simulink model "ITCG_2D_salvo_attack"  (R2023b)
settings: Solver=ode4  StartTime=0.0  StopTime=45  FixedStep=1/100  RelTol=1e-3
libraries: simulink x4, simulink_extras x1
settings Model: Creator=Administrator  LastModifiedBy=Administrator
settings DebuggingCC: UnderSpecifiedDimensionMsg=warning

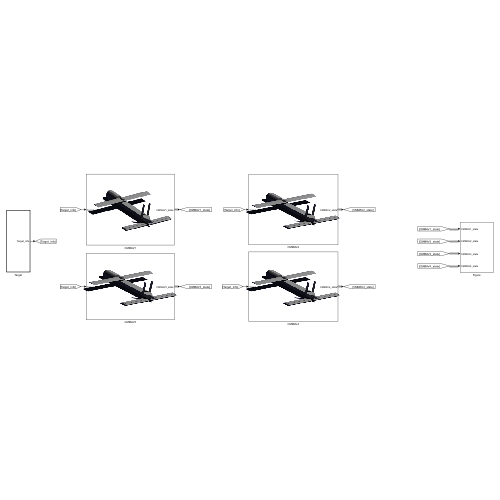
[thumbnail: Simulink's stored preview of the top-level diagram]
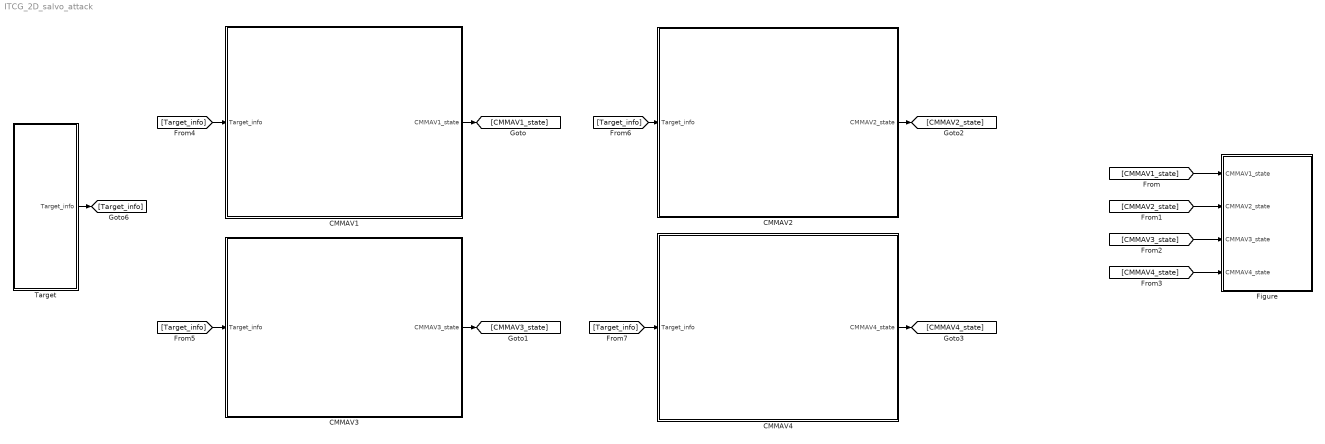
== system ITCG_2D_salvo_attack ==
  CMMAV1 : Subsystem
      mask Display: image('그림5.svg');
  CMMAV2 : Subsystem
  CMMAV3 : Subsystem
  CMMAV4 : Subsystem
  Figure : Subsystem
  Target : Subsystem  TreatAsAtomicUnit=on
  wires:
  [CMMAV1_state] -> Figure/1(CMMAV1_state)
  CMMAV1/1(CMMAV1_state) -> [CMMAV1_state]
  CMMAV3/1(CMMAV3_state) -> [CMMAV3_state]
  CMMAV2/1(CMMAV2_state) -> [CMMAV2_state]
  CMMAV4/1(CMMAV4_state) -> [CMMAV4_state]
  [CMMAV2_state] -> Figure/2(CMMAV2_state)
  [CMMAV3_state] -> Figure/3(CMMAV3_state)
  [CMMAV4_state] -> Figure/4(CMMAV4_state)
  Target/1(Target_info) -> [Target_info]
  [Target_info] -> CMMAV1/1(Target_info)
  [Target_info] -> CMMAV3/1(Target_info)
  [Target_info] -> CMMAV2/1(Target_info)
  [Target_info] -> CMMAV4/1(Target_info)

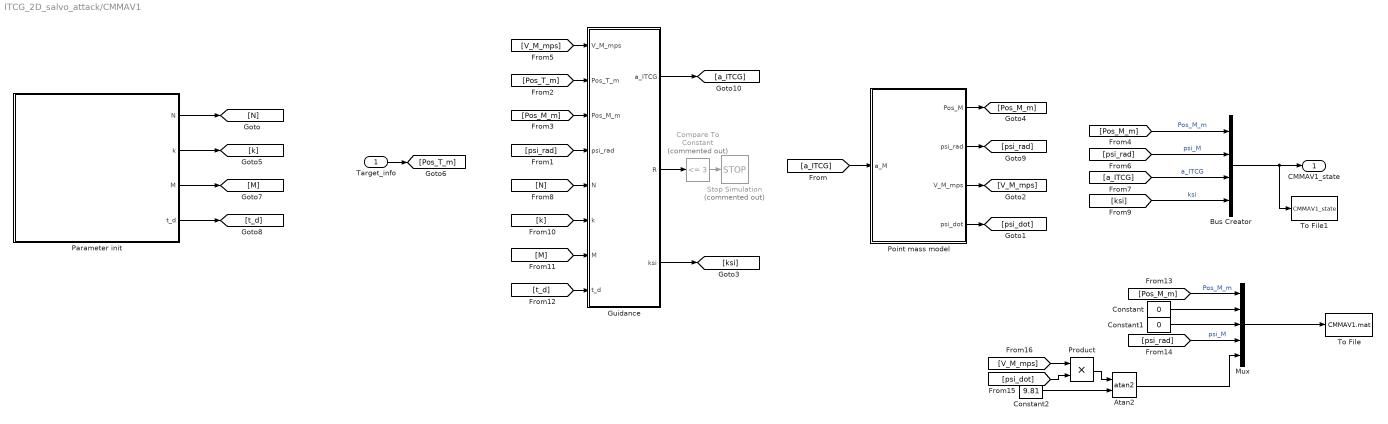
== system ITCG_2D_salvo_attack/CMMAV1 ==
  Target_info : Inport
  Atan2 : Trigonometry  Operator=atan2
  Bus Creator : BusCreator  Inputs=4
  Compare To Constant : simulink/Logic and Bit Operations/Compare To Constant  Commented=on  relop=<=  const=3  OutDataTypeStr=boolean
  Constant : Constant  Value=0
  Constant1 : Constant  Value=0
  Constant2 : Constant  Value=9.81
  Guidance : Subsystem
  Mux : Mux  Inputs=5
  Parameter init : Subsystem
  Point mass model : Subsystem
  Product : Product
  Stop Simulation : Stop  Commented=on
  To File : ToFile  Filename=CMMAV1.mat
  To File1 : ToFile  Filename=CMMAV1_state
  CMMAV1_state : Outport
  wires:
  Point mass model/2(psi_rad) -> [psi_rad]
  [M] -> Guidance/7(M)
  [k] -> Guidance/6(k)
  [Pos_M_m] -> Guidance/3(Pos_M_m)
  Target_info/1 -> [Pos_T_m]
  [N] -> Guidance/5(N)
  [a_ITCG] -> Point mass model/1(a_M)
  [Pos_T_m] -> Guidance/2(Pos_T_m)
  Guidance/2(R) -> Compare To Constant/1
  Point mass model/1(Pos_M) -> [Pos_M_m]
  [V_M_mps] -> Guidance/1(V_M_mps)
  [t_d] -> Guidance/8(t_d)
  Compare To Constant/1 -> Stop Simulation/1
  [psi_rad] -> Guidance/4(psi_rad)
  Guidance/1(a_ITCG) -> [a_ITCG]
  Point mass model/3(V_M_mps) -> [V_M_mps]
  Guidance/3(ksi) -> [ksi]
  Parameter init/3(M) -> [M]
  Parameter init/4(t_d) -> [t_d]
  Parameter init/2(k) -> [k]
  Parameter init/1(N) -> [N]
  [Pos_M_m] -> Bus Creator/1  "Pos_M_m"
  [psi_rad] -> Bus Creator/2  "psi_M"
  [a_ITCG] -> Bus Creator/3  "a_ITCG"
  [ksi] -> Bus Creator/4  "ksi"
  Bus Creator/1 -> To File1/1, CMMAV1_state/1
  [Pos_M_m] -> Mux/1  "Pos_M_m"
  Constant/1 -> Mux/2
  Constant1/1 -> Mux/3
  Point mass model/4(psi_dot) -> [psi_dot]
  Constant2/1 -> Atan2/2
  [psi_dot] -> Product/2
  [V_M_mps] -> Product/1
  Product/1 -> Atan2/1
  Atan2/1 -> Mux/5
  Mux/1 -> To File/1
  [psi_rad] -> Mux/4  "psi_M"

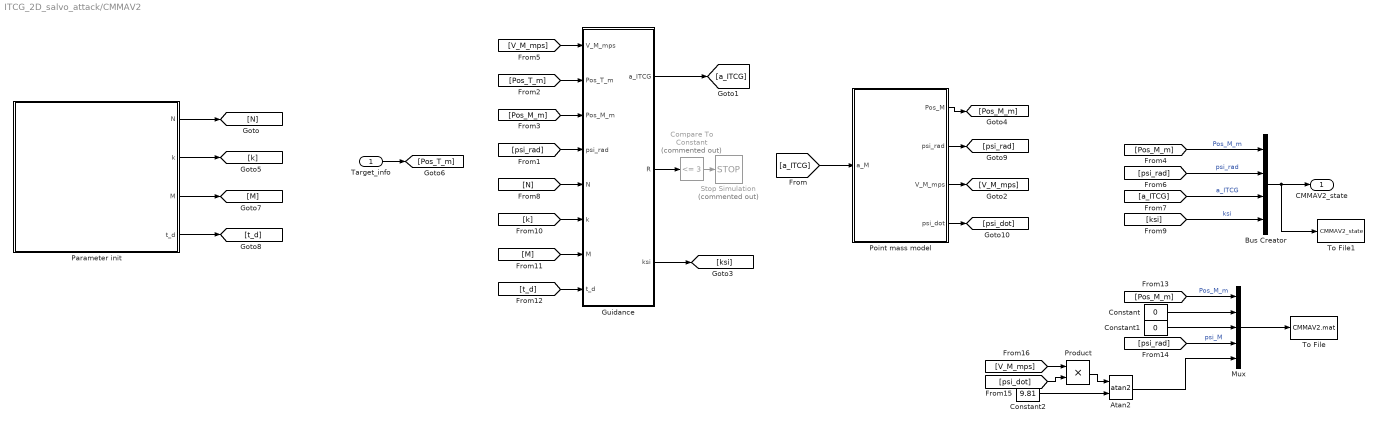
== system ITCG_2D_salvo_attack/CMMAV2 ==
  Target_info : Inport
  Atan2 : Trigonometry  Operator=atan2
  Bus Creator : BusCreator  Inputs=4
  Compare To Constant : simulink/Logic and Bit Operations/Compare To Constant  Commented=on  relop=<=  const=3  OutDataTypeStr=boolean
  Constant : Constant  Value=0
  Constant1 : Constant  Value=0
  Constant2 : Constant  Value=9.81
  Guidance : Subsystem
  Mux : Mux  Inputs=5
  Parameter init : Subsystem
  Point mass model : Subsystem
  Product : Product
  Stop Simulation : Stop  Commented=on
  To File : ToFile  Filename=CMMAV2.mat
  To File1 : ToFile  Filename=CMMAV2_state
  CMMAV2_state : Outport
  wires:
  Point mass model/2(psi_rad) -> [psi_rad]
  [M] -> Guidance/7(M)
  [k] -> Guidance/6(k)
  [Pos_M_m] -> Guidance/3(Pos_M_m)
  [N] -> Guidance/5(N)
  [a_ITCG] -> Point mass model/1(a_M)
  [Pos_T_m] -> Guidance/2(Pos_T_m)
  Guidance/2(R) -> Compare To Constant/1
  Point mass model/1(Pos_M) -> [Pos_M_m]
  [V_M_mps] -> Guidance/1(V_M_mps)
  [t_d] -> Guidance/8(t_d)
  Compare To Constant/1 -> Stop Simulation/1
  [psi_rad] -> Guidance/4(psi_rad)
  Guidance/1(a_ITCG) -> [a_ITCG]
  Point mass model/3(V_M_mps) -> [V_M_mps]
  Guidance/3(ksi) -> [ksi]
  Parameter init/1(N) -> [N]
  Parameter init/2(k) -> [k]
  Parameter init/3(M) -> [M]
  Parameter init/4(t_d) -> [t_d]
  [psi_rad] -> Bus Creator/2  "psi_rad"
  [ksi] -> Bus Creator/4  "ksi"
  [Pos_M_m] -> Bus Creator/1  "Pos_M_m"
  [a_ITCG] -> Bus Creator/3  "a_ITCG"
  Mux/1 -> To File/1
  [V_M_mps] -> Product/1
  Constant2/1 -> Atan2/2
  Product/1 -> Atan2/1
  Atan2/1 -> Mux/5
  Constant1/1 -> Mux/3
  [psi_rad] -> Mux/4  "psi_M"
  Constant/1 -> Mux/2
  [psi_dot] -> Product/2
  [Pos_M_m] -> Mux/1  "Pos_M_m"
  Point mass model/4(psi_dot) -> [psi_dot]
  Target_info/1 -> [Pos_T_m]
  Bus Creator/1 -> To File1/1, CMMAV2_state/1

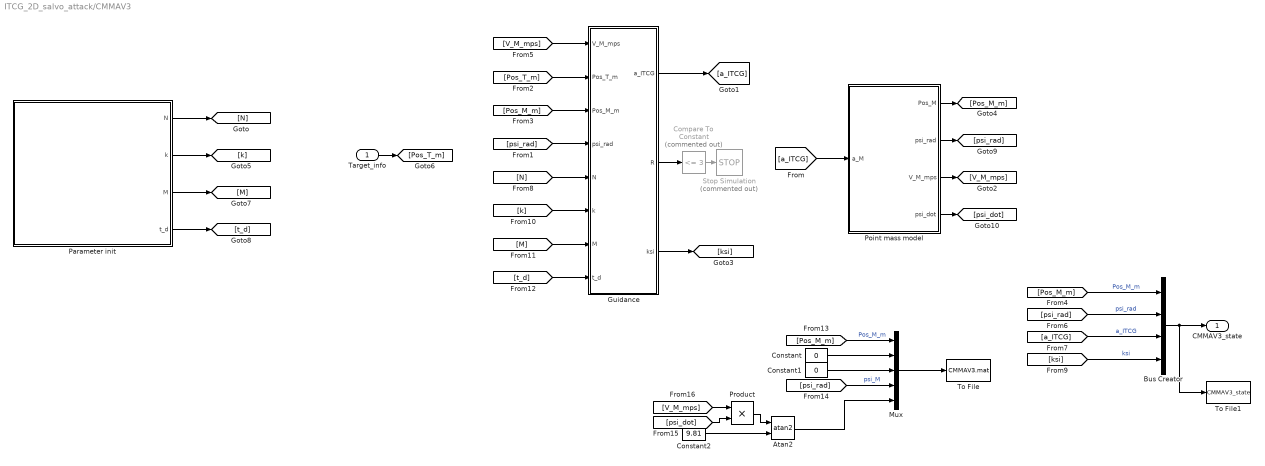
== system ITCG_2D_salvo_attack/CMMAV3 ==
  Target_info : Inport
  Atan2 : Trigonometry  Operator=atan2
  Bus Creator : BusCreator  Inputs=4
  Compare To Constant : simulink/Logic and Bit Operations/Compare To Constant  Commented=on  relop=<=  const=3  OutDataTypeStr=boolean
  Constant : Constant  Value=0
  Constant1 : Constant  Value=0
  Constant2 : Constant  Value=9.81
  Guidance : Subsystem
  Mux : Mux  Inputs=5
  Parameter init : Subsystem
  Point mass model : Subsystem
  Product : Product
  Stop Simulation : Stop  Commented=on
  To File : ToFile  Filename=CMMAV3.mat
  To File1 : ToFile  Filename=CMMAV3_state
  CMMAV3_state : Outport
  wires:
  Point mass model/2(psi_rad) -> [psi_rad]
  [M] -> Guidance/7(M)
  [k] -> Guidance/6(k)
  [Pos_M_m] -> Guidance/3(Pos_M_m)
  Target_info/1 -> [Pos_T_m]
  [N] -> Guidance/5(N)
  [a_ITCG] -> Point mass model/1(a_M)
  [Pos_T_m] -> Guidance/2(Pos_T_m)
  Guidance/2(R) -> Compare To Constant/1
  Point mass model/1(Pos_M) -> [Pos_M_m]
  [V_M_mps] -> Guidance/1(V_M_mps)
  [t_d] -> Guidance/8(t_d)
  Compare To Constant/1 -> Stop Simulation/1
  [psi_rad] -> Guidance/4(psi_rad)
  Guidance/1(a_ITCG) -> [a_ITCG]
  Point mass model/3(V_M_mps) -> [V_M_mps]
  Guidance/3(ksi) -> [ksi]
  Parameter init/1(N) -> [N]
  Parameter init/2(k) -> [k]
  Parameter init/3(M) -> [M]
  Parameter init/4(t_d) -> [t_d]
  [psi_rad] -> Bus Creator/2  "psi_rad"
  [ksi] -> Bus Creator/4  "ksi"
  [Pos_M_m] -> Bus Creator/1  "Pos_M_m"
  [a_ITCG] -> Bus Creator/3  "a_ITCG"
  Mux/1 -> To File/1
  [V_M_mps] -> Product/1
  Constant2/1 -> Atan2/2
  Product/1 -> Atan2/1
  Atan2/1 -> Mux/5
  Constant1/1 -> Mux/3
  [psi_rad] -> Mux/4  "psi_M"
  Constant/1 -> Mux/2
  [psi_dot] -> Product/2
  [Pos_M_m] -> Mux/1  "Pos_M_m"
  Point mass model/4(psi_dot) -> [psi_dot]
  Bus Creator/1 -> CMMAV3_state/1, To File1/1

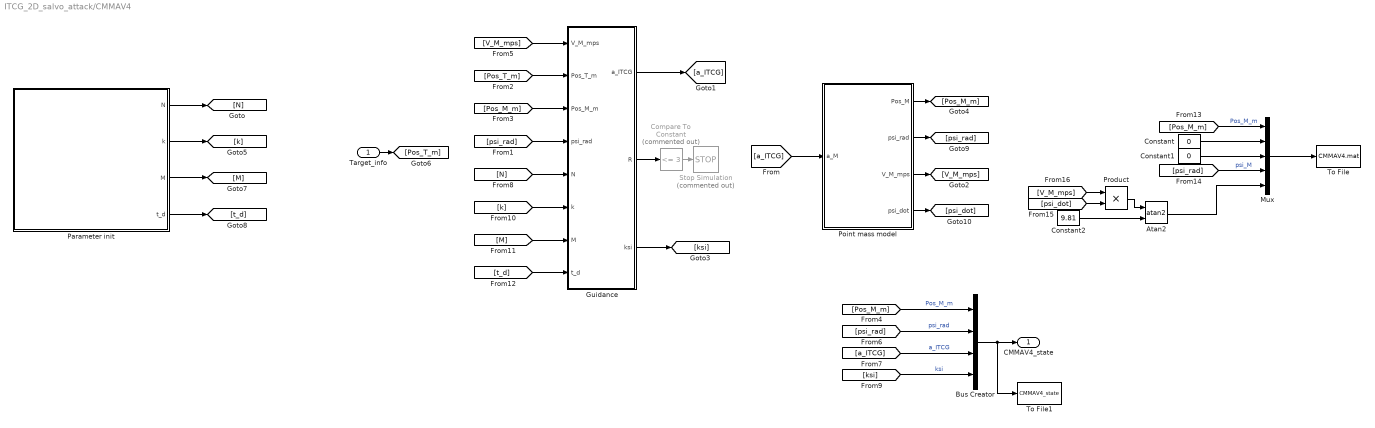
== system ITCG_2D_salvo_attack/CMMAV4 ==
  Target_info : Inport
  Atan2 : Trigonometry  Operator=atan2
  Bus Creator : BusCreator  Inputs=4
  Compare To Constant : simulink/Logic and Bit Operations/Compare To Constant  Commented=on  relop=<=  const=3  OutDataTypeStr=boolean
  Constant : Constant  Value=0
  Constant1 : Constant  Value=0
  Constant2 : Constant  Value=9.81
  Guidance : Subsystem
  Mux : Mux  Inputs=5
  Parameter init : Subsystem
  Point mass model : Subsystem
  Product : Product
  Stop Simulation : Stop  Commented=on
  To File : ToFile  Filename=CMMAV4.mat
  To File1 : ToFile  Filename=CMMAV4_state
  CMMAV4_state : Outport
  wires:
  Point mass model/2(psi_rad) -> [psi_rad]
  [M] -> Guidance/7(M)
  [k] -> Guidance/6(k)
  [Pos_M_m] -> Guidance/3(Pos_M_m)
  Target_info/1 -> [Pos_T_m]
  [N] -> Guidance/5(N)
  [a_ITCG] -> Point mass model/1(a_M)
  [Pos_T_m] -> Guidance/2(Pos_T_m)
  Guidance/2(R) -> Compare To Constant/1
  Point mass model/1(Pos_M) -> [Pos_M_m]
  [V_M_mps] -> Guidance/1(V_M_mps)
  [t_d] -> Guidance/8(t_d)
  Compare To Constant/1 -> Stop Simulation/1
  [psi_rad] -> Guidance/4(psi_rad)
  Guidance/1(a_ITCG) -> [a_ITCG]
  Point mass model/3(V_M_mps) -> [V_M_mps]
  Guidance/3(ksi) -> [ksi]
  Parameter init/1(N) -> [N]
  Parameter init/2(k) -> [k]
  Parameter init/3(M) -> [M]
  Parameter init/4(t_d) -> [t_d]
  [psi_rad] -> Bus Creator/2  "psi_rad"
  [ksi] -> Bus Creator/4  "ksi"
  [Pos_M_m] -> Bus Creator/1  "Pos_M_m"
  [a_ITCG] -> Bus Creator/3  "a_ITCG"
  Mux/1 -> To File/1
  [V_M_mps] -> Product/1
  Constant2/1 -> Atan2/2
  Product/1 -> Atan2/1
  Atan2/1 -> Mux/5
  Constant1/1 -> Mux/3
  [psi_rad] -> Mux/4  "psi_M"
  Constant/1 -> Mux/2
  [psi_dot] -> Product/2
  [Pos_M_m] -> Mux/1  "Pos_M_m"
  Point mass model/4(psi_dot) -> [psi_dot]
  Bus Creator/1 -> To File1/1, CMMAV4_state/1

== system ITCG_2D_salvo_attack/Figure ==
  note: Figure
  note: Input parameter
  CMMAV1_state : Inport
  CMMAV2_state : Inport  Port=2
  CMMAV3_state : Inport  Port=3
  CMMAV4_state : Inport  Port=4
  Bus Selector{,1..3} (4 alike) : BusSelector  OutputSignals=Pos_M_m
  Demux{1..4} (4 alike) : Demux  Outputs=2
  Figure : MATLAB Function  TreatAsAtomicUnit=on
  To Workspace : ToWorkspace  VariableName=CMMAV1_state  SampleTime=-1
  To Workspace1 : ToWorkspace  VariableName=CMMAV2_state  SampleTime=-1
  To Workspace2 : ToWorkspace  VariableName=CMMAV3_state  SampleTime=-1
  To Workspace3 : ToWorkspace  VariableName=CMMAV4_state  SampleTime=-1
  wires:
  [CMMAV1_x] -> Figure/1(CMMAV1_x)
  [CMMAV1_y] -> Figure/2(CMMAV1_y)
  [CMMAV2_x] -> Figure/3(CMMAV2_x)
  [CMMAV2_y] -> Figure/4(CMMAV2_y)
  CMMAV1_state/1 -> Bus Selector/1
  Bus Selector/1 -> To Workspace/1, Demux1/1  "<Pos_M_m>"
  Demux1/1 -> [CMMAV1_x]
  Demux1/2 -> [CMMAV1_y]
  Demux2/1 -> [CMMAV2_x]
  Demux2/2 -> [CMMAV2_y]
  Bus Selector1/1 -> To Workspace1/1, Demux2/1  "<Pos_M_m>"
  CMMAV2_state/1 -> Bus Selector1/1
  Demux3/1 -> [CMMAV3_x]
  Demux3/2 -> [CMMAV3_y]
  Bus Selector2/1 -> To Workspace2/1, Demux3/1  "<Pos_M_m>"
  CMMAV3_state/1 -> Bus Selector2/1
  Demux4/1 -> [CMMAV4_x]
  Demux4/2 -> [CMMAV4_y]
  Bus Selector3/1 -> To Workspace3/1, Demux4/1  "<Pos_M_m>"
  CMMAV4_state/1 -> Bus Selector3/1
  [CMMAV3_x] -> Figure/5(CMMAV3_x)
  [CMMAV3_y] -> Figure/6(CMMAV3_y)
  [CMMAV4_x] -> Figure/7(CMMAV4_x)
  [CMMAV4_y] -> Figure/8(CMMAV4_y)

== system ITCG_2D_salvo_attack/Target ==
  Add : Sum
  Add1 : Sum
  Demux : Demux  Outputs=2
  Demux1 : Demux  Outputs=2
  Integrator : Integrator
  Integrator1 : Integrator
  Mux1 : Mux  Inputs=2
  Target Position : Constant  Value=[00;00]  VectorParams1D=off
  Target Velocity : Constant  Value=[0;0]  VectorParams1D=off
  Target_info : Outport
  wires:
  Target Velocity/1 -> Demux/1
  Target Position/1 -> Demux1/1
  Add/1 -> Mux1/1
  Add1/1 -> Mux1/2
  Mux1/1 -> Target_info/1
  Demux1/1 -> [rT_x]
  [rT_x] -> Add/1
  Demux1/2 -> [rT_Y]
  [rT_Y] -> Add1/1
  Demux/1 -> [vT_x]
  Demux/2 -> [rT_y]
  [vT_xt] -> Add/2
  [vT_yt] -> Add1/2
  [vT_x] -> Integrator/1
  [rT_y] -> Integrator1/1
  Integrator/1 -> [vT_xt]
  Integrator1/1 -> [vT_yt]

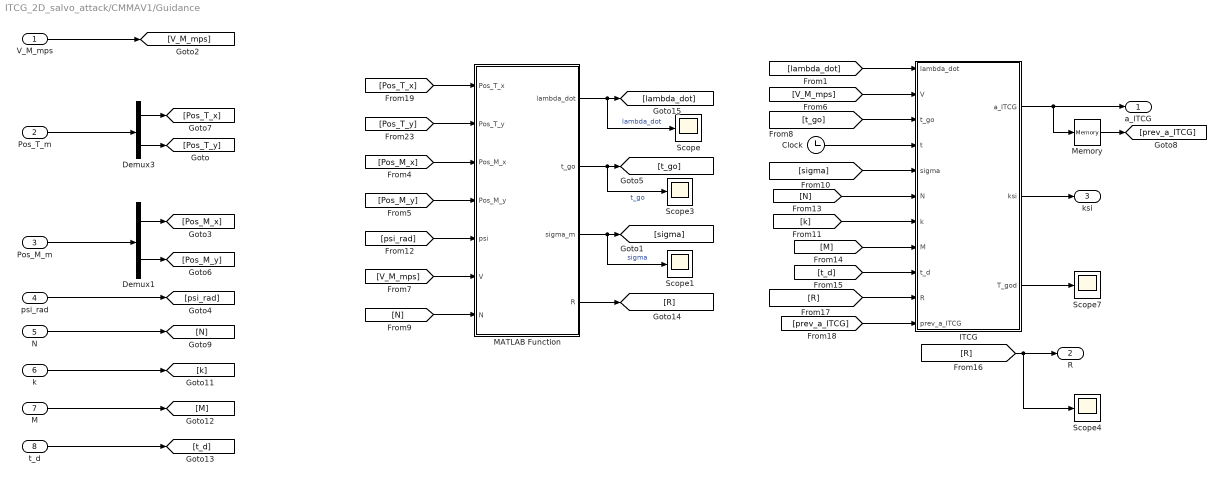
== system ITCG_2D_salvo_attack/CMMAV1/Guidance ==
  V_M_mps : Inport
  Pos_T_m : Inport  Port=2
  Pos_M_m : Inport  Port=3
  psi_rad : Inport  Port=4
  N : Inport  Port=5
  k : Inport  Port=6
  M : Inport  Port=7
  t_d : Inport  Port=8
  Clock : Clock
  Demux1 : Demux  Outputs=2
  Demux3 : Demux  Outputs=2
  ITCG : MATLAB Function  TreatAsAtomicUnit=on
  MATLAB Function : MATLAB Function  TreatAsAtomicUnit=on
  Memory : Memory
  Scope{,1,3..4,7} (5 alike) : Scope
  a_ITCG : Outport
  R : Outport  Port=2
  ksi : Outport  Port=3
  wires:
  ITCG/1(a_ITCG) -> Memory/1, a_ITCG/1
  V_M_mps/1 -> [V_M_mps]
  [V_M_mps] -> ITCG/2(V)
  [lambda_dot] -> ITCG/1(lambda_dot)
  [V_M_mps] -> MATLAB Function/6(V)
  psi_rad/1 -> [psi_rad]
  Pos_T_m/1 -> Demux3/1
  Demux3/1 -> [Pos_T_x]
  Demux1/2 -> [Pos_M_y]
  Pos_M_m/1 -> Demux1/1
  Demux1/1 -> [Pos_M_x]
  Demux3/2 -> [Pos_T_y]
  MATLAB Function/1(lambda_dot) -> [lambda_dot], Scope/1  "lambda_dot"
  MATLAB Function/2(t_go) -> Scope3/1, [t_go]  "t_go"
  Clock/1 -> ITCG/4(t)
  [Pos_M_x] -> MATLAB Function/3(Pos_M_x)
  [Pos_M_y] -> MATLAB Function/4(Pos_M_y)
  [Pos_T_x] -> MATLAB Function/1(Pos_T_x)
  [Pos_T_y] -> MATLAB Function/2(Pos_T_y)
  [psi_rad] -> MATLAB Function/5(psi)
  MATLAB Function/3(sigma_m) -> Scope1/1, [sigma]  "sigma"
  [t_go] -> ITCG/3(t_go)
  [sigma] -> ITCG/5(sigma)
  ITCG/2(ksi) -> ksi/1
  N/1 -> [N]
  t_d/1 -> [t_d]
  M/1 -> [M]
  k/1 -> [k]
  [N] -> MATLAB Function/7(N)
  [N] -> ITCG/6(N)
  [k] -> ITCG/7(k)
  [M] -> ITCG/8(M)
  [t_d] -> ITCG/9(t_d)
  MATLAB Function/4(R) -> [R]
  [R] -> Scope4/1, R/1
  [R] -> ITCG/10(R)
  Memory/1 -> [prev_a_ITCG]
  [prev_a_ITCG] -> ITCG/11(prev_a_ITCG)
  ITCG/3(T_god) -> Scope7/1

== system ITCG_2D_salvo_attack/CMMAV1/Parameter init ==
  Constant : Constant  Value=3
  Constant1 : Constant  Value=2
  Constant2 : Constant  Value=10
  Constant3 : Constant  Value=30
  N : Outport
  k : Outport  Port=2
  M : Outport  Port=3
  t_d : Outport  Port=4
  wires:
  Constant/1 -> N/1
  Constant1/1 -> k/1
  Constant2/1 -> M/1
  Constant3/1 -> t_d/1

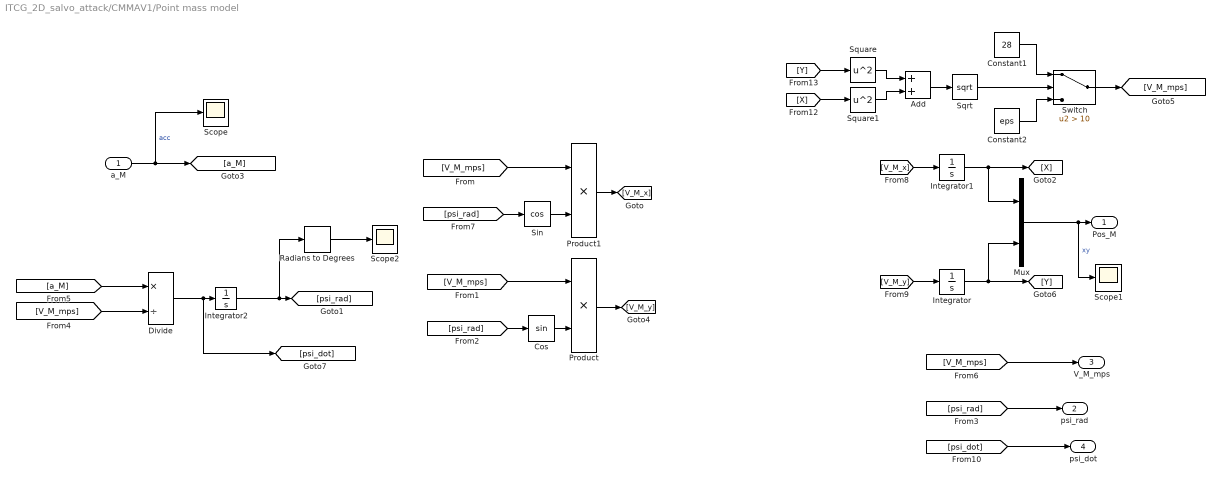
== system ITCG_2D_salvo_attack/CMMAV1/Point mass model ==
  a_M : Inport
  Add : Sum
  Constant1 : Constant  Value=28
  Constant2 : Constant  Value=eps
  Cos : Trigonometry
  Divide : Product  Inputs=*/
  Integrator : Integrator  InitialCondition=500
  Integrator1 : Integrator  InitialCondition=300
  Integrator2 : Integrator  InitialCondition=0*pi/180
  Mux : Mux  Inputs=2
  Product : Product
  Product1 : Product
  Radians to Degrees : simulink_extras/Transformations/Radians to Degrees
  Scope : Scope
  Scope1 : Scope
  Scope2 : Scope
  Sin : Trigonometry  Operator=cos
  Sqrt : Sqrt
  Square : Math  Operator=square
  Square1 : Math  Operator=square
  Switch : Switch  Criteria=u2 > Threshold  Threshold=10  SaturateOnIntegerOverflow=off  InputSameDT=off
  Pos_M : Outport
  psi_rad : Outport  Port=2
  V_M_mps : Outport  Port=3
  psi_dot : Outport  Port=4
  wires:
  [V_M_mps] -> Product1/1
  [V_M_mps] -> Product/1
  [psi_rad] -> Sin/1
  [psi_rad] -> Cos/1
  Cos/1 -> Product/2
  Sin/1 -> Product1/2
  Mux/1 -> Scope1/1, Pos_M/1  "xy"
  [psi_rad] -> psi_rad/1
  Integrator/1 -> [Y], Mux/2
  Integrator1/1 -> [X], Mux/1
  Divide/1 -> [psi_dot], Integrator2/1
  [V_M_mps] -> Divide/2
  [V_M_mps] -> V_M_mps/1
  [a_M] -> Divide/1
  a_M/1 -> Scope/1, [a_M]  "acc"
  Product1/1 -> [V_M_x]
  Product/1 -> [V_M_y]
  [V_M_x] -> Integrator1/1
  [V_M_y] -> Integrator/1
  Integrator2/1 -> Radians to Degrees/1, [psi_rad]
  Switch/1 -> [V_M_mps]
  [Y] -> Square/1
  Square1/1 -> Add/2
  Constant1/1 -> Switch/1
  Square/1 -> Add/1
  [X] -> Square1/1
  Sqrt/1 -> Switch/2
  Add/1 -> Sqrt/1
  Constant2/1 -> Switch/3
  [psi_dot] -> psi_dot/1
  Radians to Degrees/1 -> Scope2/1

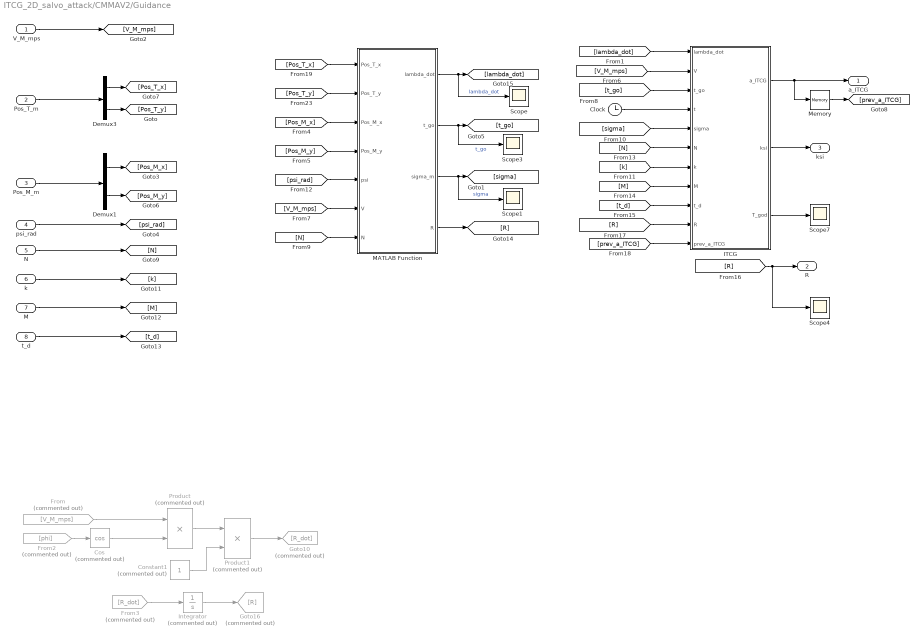
== system ITCG_2D_salvo_attack/CMMAV2/Guidance ==
  V_M_mps : Inport
  Pos_T_m : Inport  Port=2
  Pos_M_m : Inport  Port=3
  psi_rad : Inport  Port=4
  N : Inport  Port=5
  k : Inport  Port=6
  M : Inport  Port=7
  t_d : Inport  Port=8
  Clock : Clock
  Constant1 : Constant  Commented=on
  Cos : Trigonometry  Commented=on  Operator=cos
  Demux1 : Demux  Outputs=2
  Demux3 : Demux  Outputs=2
  From : From  Commented=on  GotoTag=V_M_mps
  From2 : From  Commented=on  GotoTag=phi
  From3 : From  Commented=on  GotoTag=R_dot
  Goto10 : Goto  Commented=on  GotoTag=R_dot
  Goto16 : Goto  Commented=on  GotoTag=R
  ITCG : MATLAB Function  TreatAsAtomicUnit=on
  Integrator : Integrator  Commented=on
  MATLAB Function : MATLAB Function  TreatAsAtomicUnit=on
  Memory : Memory
  Product : Product  Commented=on
  Product1 : Product  Commented=on
  Scope{,1,3..4,7} (5 alike) : Scope
  a_ITCG : Outport
  R : Outport  Port=2
  ksi : Outport  Port=3
  wires:
  ITCG/1(a_ITCG) -> Memory/1, a_ITCG/1
  V_M_mps/1 -> [V_M_mps]
  [V_M_mps] -> ITCG/2(V)
  [lambda_dot] -> ITCG/1(lambda_dot)
  [V_M_mps] -> MATLAB Function/6(V)
  psi_rad/1 -> [psi_rad]
  Pos_T_m/1 -> Demux3/1
  Demux3/1 -> [Pos_T_x]
  Demux1/2 -> [Pos_M_y]
  Pos_M_m/1 -> Demux1/1
  Demux1/1 -> [Pos_M_x]
  Demux3/2 -> [Pos_T_y]
  MATLAB Function/1(lambda_dot) -> [lambda_dot], Scope/1  "lambda_dot"
  MATLAB Function/2(t_go) -> Scope3/1, [t_go]  "t_go"
  Clock/1 -> ITCG/4(t)
  From2/1 -> Cos/1
  From/1 -> Product/1
  Cos/1 -> Product/2
  Product/1 -> Product1/1
  Constant1/1 -> Product1/2
  Product1/1 -> Goto10/1
  From3/1 -> Integrator/1
  Integrator/1 -> Goto16/1
  [Pos_M_x] -> MATLAB Function/3(Pos_M_x)
  [Pos_M_y] -> MATLAB Function/4(Pos_M_y)
  [Pos_T_x] -> MATLAB Function/1(Pos_T_x)
  [Pos_T_y] -> MATLAB Function/2(Pos_T_y)
  [psi_rad] -> MATLAB Function/5(psi)
  MATLAB Function/3(sigma_m) -> Scope1/1, [sigma]  "sigma"
  [t_go] -> ITCG/3(t_go)
  [sigma] -> ITCG/5(sigma)
  ITCG/2(ksi) -> ksi/1
  N/1 -> [N]
  t_d/1 -> [t_d]
  M/1 -> [M]
  k/1 -> [k]
  [N] -> MATLAB Function/7(N)
  [N] -> ITCG/6(N)
  [k] -> ITCG/7(k)
  [M] -> ITCG/8(M)
  [t_d] -> ITCG/9(t_d)
  MATLAB Function/4(R) -> [R]
  [R] -> Scope4/1, R/1
  [R] -> ITCG/10(R)
  Memory/1 -> [prev_a_ITCG]
  [prev_a_ITCG] -> ITCG/11(prev_a_ITCG)
  ITCG/3(T_god) -> Scope7/1

== system ITCG_2D_salvo_attack/CMMAV2/Parameter init ==
  Constant : Constant  Value=3
  Constant1 : Constant  Value=2
  Constant2 : Constant  Value=10
  Constant3 : Constant  Value=35
  N : Outport
  k : Outport  Port=2
  M : Outport  Port=3
  t_d : Outport  Port=4
  wires:
  Constant3/1 -> t_d/1
  Constant1/1 -> k/1
  Constant2/1 -> M/1
  Constant/1 -> N/1

== system ITCG_2D_salvo_attack/CMMAV2/Point mass model ==
  a_M : Inport
  Add : Sum
  Constant : Constant  Value=28
  Constant1 : Constant  Value=eps
  Cos : Trigonometry
  Divide : Product  Inputs=*/
  Integrator : Integrator  InitialCondition=500
  Integrator1 : Integrator  InitialCondition=-300
  Integrator2 : Integrator  InitialCondition=90*pi/180
  Mux : Mux  Inputs=2
  Product : Product
  Product1 : Product
  Sin : Trigonometry  Operator=cos
  Sqrt : Sqrt
  Square : Math  Operator=square
  Square1 : Math  Operator=square
  Switch : Switch  Criteria=u2 > Threshold  Threshold=10  SaturateOnIntegerOverflow=off  InputSameDT=off
  Pos_M : Outport
  psi_rad : Outport  Port=2
  V_M_mps : Outport  Port=3
  psi_dot : Outport  Port=4
  wires:
  [V_M_mps] -> Product1/1
  [V_M_mps] -> Product/1
  [psi_rad] -> Sin/1
  [psi_rad] -> Cos/1
  Cos/1 -> Product/2
  Sin/1 -> Product1/2
  Mux/1 -> Pos_M/1
  [psi_rad] -> psi_rad/1
  Integrator/1 -> [Y]
  Integrator1/1 -> [X]
  Divide/1 -> psi_dot/1, Integrator2/1
  [V_M_mps] -> Divide/2
  [V_M_mps] -> V_M_mps/1
  [a_M] -> Divide/1
  a_M/1 -> [a_M]
  Product1/1 -> [V_M_x]
  Product/1 -> [V_M_y]
  [V_M_x] -> Integrator1/1
  [V_M_y] -> Integrator/1
  Integrator2/1 -> [psi_rad]
  [Y] -> Square/1
  [X] -> Square1/1
  Square/1 -> Add/1
  Square1/1 -> Add/2
  Add/1 -> Sqrt/1
  Sqrt/1 -> Switch/2
  Constant/1 -> Switch/1
  Switch/1 -> [V_M_mps]
  Constant1/1 -> Switch/3
  [Y] -> Mux/2
  [X] -> Mux/1

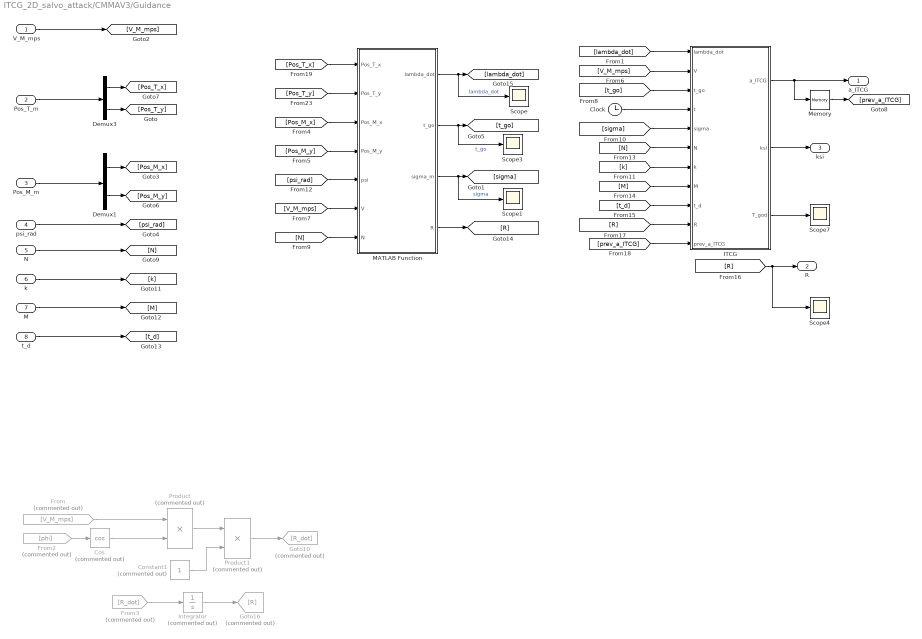
== system ITCG_2D_salvo_attack/CMMAV3/Guidance ==
  V_M_mps : Inport
  Pos_T_m : Inport  Port=2
  Pos_M_m : Inport  Port=3
  psi_rad : Inport  Port=4
  N : Inport  Port=5
  k : Inport  Port=6
  M : Inport  Port=7
  t_d : Inport  Port=8
  Clock : Clock
  Constant1 : Constant  Commented=on
  Cos : Trigonometry  Commented=on  Operator=cos
  Demux1 : Demux  Outputs=2
  Demux3 : Demux  Outputs=2
  From : From  Commented=on  GotoTag=V_M_mps
  From2 : From  Commented=on  GotoTag=phi
  From3 : From  Commented=on  GotoTag=R_dot
  Goto10 : Goto  Commented=on  GotoTag=R_dot
  Goto16 : Goto  Commented=on  GotoTag=R
  ITCG : MATLAB Function  TreatAsAtomicUnit=on
  Integrator : Integrator  Commented=on
  MATLAB Function : MATLAB Function  TreatAsAtomicUnit=on
  Memory : Memory
  Product : Product  Commented=on
  Product1 : Product  Commented=on
  Scope{,1,3..4,7} (5 alike) : Scope
  a_ITCG : Outport
  R : Outport  Port=2
  ksi : Outport  Port=3
  wires:
  ITCG/1(a_ITCG) -> Memory/1, a_ITCG/1
  V_M_mps/1 -> [V_M_mps]
  [V_M_mps] -> ITCG/2(V)
  [lambda_dot] -> ITCG/1(lambda_dot)
  [V_M_mps] -> MATLAB Function/6(V)
  psi_rad/1 -> [psi_rad]
  Pos_T_m/1 -> Demux3/1
  Demux3/1 -> [Pos_T_x]
  Demux1/2 -> [Pos_M_y]
  Pos_M_m/1 -> Demux1/1
  Demux1/1 -> [Pos_M_x]
  Demux3/2 -> [Pos_T_y]
  MATLAB Function/1(lambda_dot) -> [lambda_dot], Scope/1  "lambda_dot"
  MATLAB Function/2(t_go) -> Scope3/1, [t_go]  "t_go"
  Clock/1 -> ITCG/4(t)
  From2/1 -> Cos/1
  From/1 -> Product/1
  Cos/1 -> Product/2
  Product/1 -> Product1/1
  Constant1/1 -> Product1/2
  Product1/1 -> Goto10/1
  From3/1 -> Integrator/1
  Integrator/1 -> Goto16/1
  [Pos_M_x] -> MATLAB Function/3(Pos_M_x)
  [Pos_M_y] -> MATLAB Function/4(Pos_M_y)
  [Pos_T_x] -> MATLAB Function/1(Pos_T_x)
  [Pos_T_y] -> MATLAB Function/2(Pos_T_y)
  [psi_rad] -> MATLAB Function/5(psi)
  MATLAB Function/3(sigma_m) -> Scope1/1, [sigma]  "sigma"
  [t_go] -> ITCG/3(t_go)
  [sigma] -> ITCG/5(sigma)
  ITCG/2(ksi) -> ksi/1
  N/1 -> [N]
  t_d/1 -> [t_d]
  M/1 -> [M]
  k/1 -> [k]
  [N] -> MATLAB Function/7(N)
  [N] -> ITCG/6(N)
  [k] -> ITCG/7(k)
  [M] -> ITCG/8(M)
  [t_d] -> ITCG/9(t_d)
  MATLAB Function/4(R) -> [R]
  [R] -> Scope4/1, R/1
  [R] -> ITCG/10(R)
  Memory/1 -> [prev_a_ITCG]
  [prev_a_ITCG] -> ITCG/11(prev_a_ITCG)
  ITCG/3(T_god) -> Scope7/1

== system ITCG_2D_salvo_attack/CMMAV3/Parameter init ==
  Constant : Constant  Value=3
  Constant1 : Constant  Value=2
  Constant2 : Constant  Value=10
  Constant3 : Constant  Value=40
  N : Outport
  k : Outport  Port=2
  M : Outport  Port=3
  t_d : Outport  Port=4
  wires:
  Constant3/1 -> t_d/1
  Constant1/1 -> k/1
  Constant2/1 -> M/1
  Constant/1 -> N/1

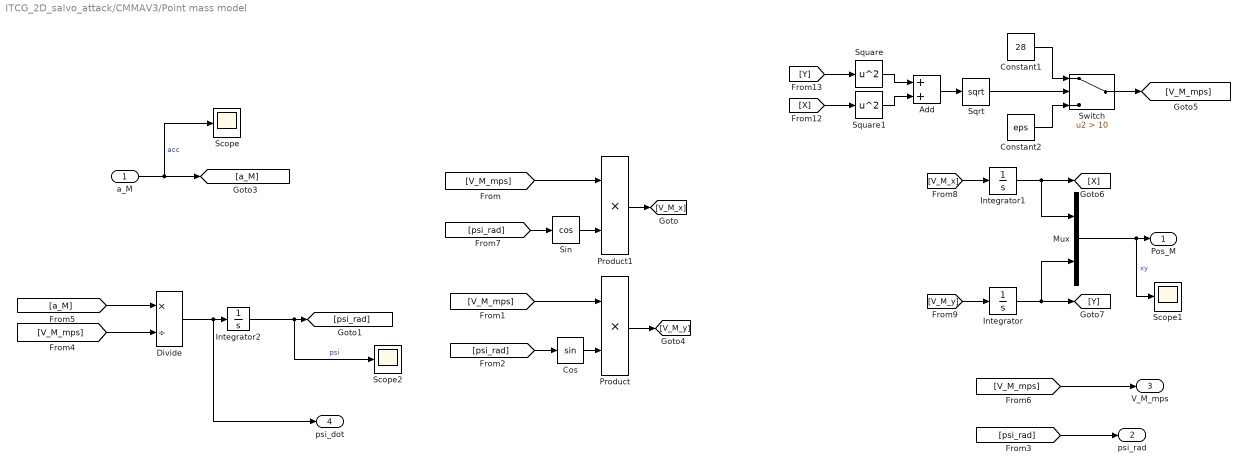
== system ITCG_2D_salvo_attack/CMMAV3/Point mass model ==
  a_M : Inport
  Add : Sum
  Constant1 : Constant  Value=28
  Constant2 : Constant  Value=eps
  Cos : Trigonometry
  Divide : Product  Inputs=*/
  Integrator : Integrator  InitialCondition=-500
  Integrator1 : Integrator  InitialCondition=300
  Integrator2 : Integrator  InitialCondition=-90*pi/180
  Mux : Mux  Inputs=2
  Product : Product
  Product1 : Product
  Scope : Scope
  Scope1 : Scope
  Scope2 : Scope
  Sin : Trigonometry  Operator=cos
  Sqrt : Sqrt
  Square : Math  Operator=square
  Square1 : Math  Operator=square
  Switch : Switch  Criteria=u2 > Threshold  Threshold=10  SaturateOnIntegerOverflow=off  InputSameDT=off
  Pos_M : Outport
  psi_rad : Outport  Port=2
  V_M_mps : Outport  Port=3
  psi_dot : Outport  Port=4
  wires:
  [V_M_mps] -> Product1/1
  [V_M_mps] -> Product/1
  [psi_rad] -> Sin/1
  [psi_rad] -> Cos/1
  Cos/1 -> Product/2
  Sin/1 -> Product1/2
  Mux/1 -> Scope1/1, Pos_M/1  "xy"
  [psi_rad] -> psi_rad/1
  Integrator/1 -> [Y], Mux/2
  Integrator1/1 -> [X], Mux/1
  Divide/1 -> psi_dot/1, Integrator2/1
  [V_M_mps] -> Divide/2
  [V_M_mps] -> V_M_mps/1
  [a_M] -> Divide/1
  a_M/1 -> Scope/1, [a_M]  "acc"
  Product1/1 -> [V_M_x]
  Product/1 -> [V_M_y]
  [V_M_x] -> Integrator1/1
  [V_M_y] -> Integrator/1
  Integrator2/1 -> Scope2/1, [psi_rad]  "psi"
  Add/1 -> Sqrt/1
  Constant2/1 -> Switch/3
  [X] -> Square1/1
  Constant1/1 -> Switch/1
  Square1/1 -> Add/2
  Sqrt/1 -> Switch/2
  Switch/1 -> [V_M_mps]
  Square/1 -> Add/1
  [Y] -> Square/1

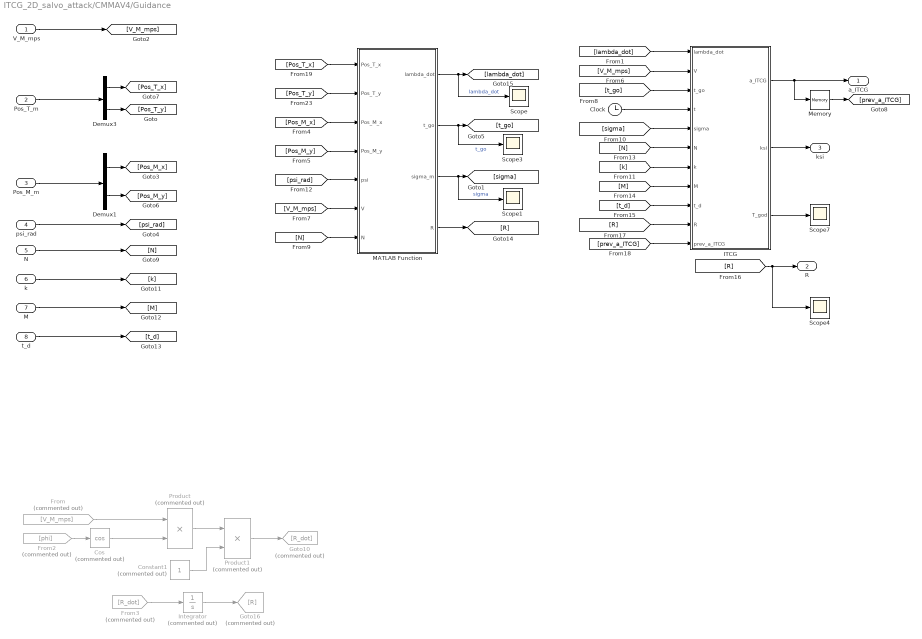
== system ITCG_2D_salvo_attack/CMMAV4/Guidance ==
  V_M_mps : Inport
  Pos_T_m : Inport  Port=2
  Pos_M_m : Inport  Port=3
  psi_rad : Inport  Port=4
  N : Inport  Port=5
  k : Inport  Port=6
  M : Inport  Port=7
  t_d : Inport  Port=8
  Clock : Clock
  Constant1 : Constant  Commented=on
  Cos : Trigonometry  Commented=on  Operator=cos
  Demux1 : Demux  Outputs=2
  Demux3 : Demux  Outputs=2
  From : From  Commented=on  GotoTag=V_M_mps
  From2 : From  Commented=on  GotoTag=phi
  From3 : From  Commented=on  GotoTag=R_dot
  Goto10 : Goto  Commented=on  GotoTag=R_dot
  Goto16 : Goto  Commented=on  GotoTag=R
  ITCG : MATLAB Function  TreatAsAtomicUnit=on
  Integrator : Integrator  Commented=on
  MATLAB Function : MATLAB Function  TreatAsAtomicUnit=on
  Memory : Memory
  Product : Product  Commented=on
  Product1 : Product  Commented=on
  Scope{,1,3..4,7} (5 alike) : Scope
  a_ITCG : Outport
  R : Outport  Port=2
  ksi : Outport  Port=3
  wires:
  ITCG/1(a_ITCG) -> Memory/1, a_ITCG/1
  V_M_mps/1 -> [V_M_mps]
  [V_M_mps] -> ITCG/2(V)
  [lambda_dot] -> ITCG/1(lambda_dot)
  [V_M_mps] -> MATLAB Function/6(V)
  psi_rad/1 -> [psi_rad]
  Pos_T_m/1 -> Demux3/1
  Demux3/1 -> [Pos_T_x]
  Demux1/2 -> [Pos_M_y]
  Pos_M_m/1 -> Demux1/1
  Demux1/1 -> [Pos_M_x]
  Demux3/2 -> [Pos_T_y]
  MATLAB Function/1(lambda_dot) -> [lambda_dot], Scope/1  "lambda_dot"
  MATLAB Function/2(t_go) -> Scope3/1, [t_go]  "t_go"
  Clock/1 -> ITCG/4(t)
  From2/1 -> Cos/1
  From/1 -> Product/1
  Cos/1 -> Product/2
  Product/1 -> Product1/1
  Constant1/1 -> Product1/2
  Product1/1 -> Goto10/1
  From3/1 -> Integrator/1
  Integrator/1 -> Goto16/1
  [Pos_M_x] -> MATLAB Function/3(Pos_M_x)
  [Pos_M_y] -> MATLAB Function/4(Pos_M_y)
  [Pos_T_x] -> MATLAB Function/1(Pos_T_x)
  [Pos_T_y] -> MATLAB Function/2(Pos_T_y)
  [psi_rad] -> MATLAB Function/5(psi)
  MATLAB Function/3(sigma_m) -> Scope1/1, [sigma]  "sigma"
  [t_go] -> ITCG/3(t_go)
  [sigma] -> ITCG/5(sigma)
  ITCG/2(ksi) -> ksi/1
  N/1 -> [N]
  t_d/1 -> [t_d]
  M/1 -> [M]
  k/1 -> [k]
  [N] -> MATLAB Function/7(N)
  [N] -> ITCG/6(N)
  [k] -> ITCG/7(k)
  [M] -> ITCG/8(M)
  [t_d] -> ITCG/9(t_d)
  MATLAB Function/4(R) -> [R]
  [R] -> Scope4/1, R/1
  [R] -> ITCG/10(R)
  Memory/1 -> [prev_a_ITCG]
  [prev_a_ITCG] -> ITCG/11(prev_a_ITCG)
  ITCG/3(T_god) -> Scope7/1

== system ITCG_2D_salvo_attack/CMMAV4/Parameter init ==
  Constant : Constant  Value=3
  Constant1 : Constant  Value=2
  Constant2 : Constant  Value=10
  Constant3 : Constant  Value=45
  N : Outport
  k : Outport  Port=2
  M : Outport  Port=3
  t_d : Outport  Port=4
  wires:
  Constant3/1 -> t_d/1
  Constant1/1 -> k/1
  Constant2/1 -> M/1
  Constant/1 -> N/1

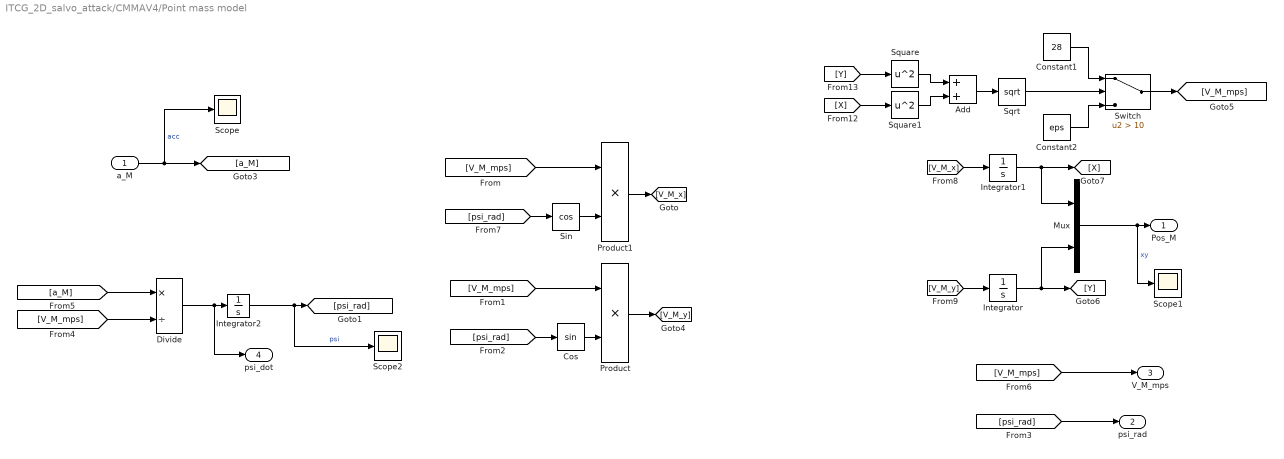
== system ITCG_2D_salvo_attack/CMMAV4/Point mass model ==
  a_M : Inport
  Add : Sum
  Constant1 : Constant  Value=28
  Constant2 : Constant  Value=eps
  Cos : Trigonometry
  Divide : Product  Inputs=*/
  Integrator : Integrator  InitialCondition=-500
  Integrator1 : Integrator  InitialCondition=-300
  Integrator2 : Integrator  InitialCondition=90*pi/180
  Mux : Mux  Inputs=2
  Product : Product
  Product1 : Product
  Scope : Scope
  Scope1 : Scope
  Scope2 : Scope
  Sin : Trigonometry  Operator=cos
  Sqrt : Sqrt
  Square : Math  Operator=square
  Square1 : Math  Operator=square
  Switch : Switch  Criteria=u2 > Threshold  Threshold=10  SaturateOnIntegerOverflow=off  InputSameDT=off
  Pos_M : Outport
  psi_rad : Outport  Port=2
  V_M_mps : Outport  Port=3
  psi_dot : Outport  Port=4
  wires:
  [V_M_mps] -> Product1/1
  [V_M_mps] -> Product/1
  [psi_rad] -> Sin/1
  [psi_rad] -> Cos/1
  Cos/1 -> Product/2
  Sin/1 -> Product1/2
  Mux/1 -> Scope1/1, Pos_M/1  "xy"
  [psi_rad] -> psi_rad/1
  Integrator/1 -> [Y], Mux/2
  Integrator1/1 -> [X], Mux/1
  Divide/1 -> psi_dot/1, Integrator2/1
  [V_M_mps] -> Divide/2
  [V_M_mps] -> V_M_mps/1
  [a_M] -> Divide/1
  a_M/1 -> Scope/1, [a_M]  "acc"
  Product1/1 -> [V_M_x]
  Product/1 -> [V_M_y]
  [V_M_x] -> Integrator1/1
  [V_M_y] -> Integrator/1
  Integrator2/1 -> Scope2/1, [psi_rad]  "psi"
  Add/1 -> Sqrt/1
  Constant2/1 -> Switch/3
  [X] -> Square1/1
  Constant1/1 -> Switch/1
  Square1/1 -> Add/2
  Sqrt/1 -> Switch/2
  Switch/1 -> [V_M_mps]
  Square/1 -> Add/1
  [Y] -> Square/1

== matlab function ITCG_2D_salvo_attack/CMMAV2/Guidance/ITCG ==
  data: a_ITCG output; lambda_dot input; V input; t_go input; t input; sigma input; ksi output; N input; k input; M input; t_d input; T_god output; R input; prev_a_ITCG input
function [a_ITCG, ksi, T_god]  = fcn(lambda_dot, V, t_go, t, sigma, N, k, M, t_d, R, prev_a_ITCG)


T_god=t_d-t;
ksi=t_go-T_god;

sgmf_ksi = 2*( (1/(1+exp(-10*ksi))) - 1/2);
% sgmf_abs_sigma = 2*( 1/(1+exp(-abs(sigma))) - 1/2);
%
%ITCG command
% a_ITCG = N*(1+k*sign(ksi))*V*theta_dot + M*(sign(abs(phi))-1)*sign(ksi);

if R <10
    a_ITCG = prev_a_ITCG;
else
    a_ITCG = N*(1+k*sgmf_ksi)*V*lambda_dot;
end



% a_ITCG = N*(1+k*sgmf_ksi)*V*lambda_dot + M*(sgmf_abs_sigma-1)*sgmf_ksi;
% function [a_ITCG, ksi, T_god]  = fcn(lambda_dot, V, t_go, t, sigma, N, k, M, t_d, R, prev_a_ITCG)
% 
% T_god = t_d-t;
% ksi = t_go-T_god;
% 
% sigma_deg = sigma * 180/pi;
% 
% sgmf_ksi = 2*( 1/(1+exp(-10*ksi)) - 1/2);
% sgmf_abs_sigma = 2*( 1/(1+exp(-10*abs(sigma_deg))) - 1/2);
% 
% a_ITCG = N*(1+k*sgmf_ksi)*V*lambda_dot + M*(sgmf_abs_sigma-1)*sgmf_ksi*0;
% 
% term = M*(sgmf_abs_sigma-1)*sgmf_ksi;
% 
% if R <10
%     a_ITCG = prev_a_ITCG;
% else
%     a_ITCG = N*(1+k*sgmf_ksi)*V*lambda_dot;
% end

== matlab function ITCG_2D_salvo_attack/CMMAV2/Guidance/MATLAB Function ==
  data: Pos_T_x input; lambda_dot output; Pos_T_y input; Pos_M_x input; Pos_M_y input; psi input; V input; N input; t_go output; sigma_m output; R output
function [lambda_dot, t_go, sigma_m, R] = fcn(Pos_T_x, Pos_T_y, Pos_M_x, Pos_M_y, psi, V, N)
    R2D=180/pi;
    D2R=pi/180;
    % relative parameter
    rTM_x = Pos_T_x - Pos_M_x;
    rTM_y = Pos_T_y - Pos_M_y;
    R=sqrt((rTM_x)^2+(rTM_y)^2);    
    lambda=atan2(rTM_y,rTM_x);
    sigma=psi-lambda;
    sigma_m=abs(mod(sigma+pi, 2*pi)-pi);
    % R_dot=-V*cos(phi);

    % a=1/(2*(N-1));
    % b=1/2;
    % 
    % B1 = integral(@(t) t.^(a-1) .* (1-t).^(b-1), 0, sin(sigma_m)^2, "AbsTol", 1e-10, "RelTol", 1e-4);
    % B2 = beta(a, b);
    % 
    % if isnan(B1)
    %     B1 = 0;
    % end
    % if isnan(B2)
    %     B2 = 0;
    % end
    % 
    % if sigma_m >= 0 && sigma_m < pi/2
    %     t_go = (R / (2*V*(N-1)*sin(sigma_m)^(1/(N-1)))) * B1;
    %     if isinf(t_go) || t_go <= 0.1
    %         t_go = 1e-3;
    %     end
    % elseif sigma_m >= pi/2 && sigma_m <= pi
    %     t_go = (R / (2*V*(N-1)*sin(sigma_m)^(1/(N-1)))) * (2*B2 - B1);
    %     if isinf(t_go) || t_go <= 0.1
    %         t_go = 1e-3;
    %     end
    % else
    %     t_go = 0;
    % end
    
    t_go = R/V*(1+(sigma_m^2/(2*(2*N-1))));

    % command
    lambda_dot = -V*sin(sigma_m)/R;

end

== matlab function ITCG_2D_salvo_attack/CMMAV3/Guidance/ITCG ==
  data: a_ITCG output; lambda_dot input; V input; t_go input; t input; sigma input; ksi output; N input; k input; M input; t_d input; T_god output; R input; prev_a_ITCG input
function [a_ITCG, ksi, T_god]  = fcn(lambda_dot, V, t_go, t, sigma, N, k, M, t_d, R, prev_a_ITCG)


T_god=t_d-t;
ksi=t_go-T_god;

sgmf_ksi = 2*( (1/(1+exp(-10*ksi))) - 1/2);
% sgmf_abs_sigma = 2*( 1/(1+exp(-abs(sigma))) - 1/2);
%
%ITCG command
% a_ITCG = N*(1+k*sign(ksi))*V*theta_dot + M*(sign(abs(phi))-1)*sign(ksi);

if R <10
    a_ITCG = prev_a_ITCG;
else
    a_ITCG = N*(1+k*sgmf_ksi)*V*lambda_dot;
end



% a_ITCG = N*(1+k*sgmf_ksi)*V*lambda_dot + M*(sgmf_abs_sigma-1)*sgmf_ksi;
% function [a_ITCG, ksi, T_god]  = fcn(lambda_dot, V, t_go, t, sigma, N, k, M, t_d, R, prev_a_ITCG)
% 
% T_god = t_d-t;
% ksi = t_go-T_god;
% 
% sigma_deg = sigma * 180/pi;
% 
% sgmf_ksi = 2*( 1/(1+exp(-10*ksi)) - 1/2);
% sgmf_abs_sigma = 2*( 1/(1+exp(-10*abs(sigma_deg))) - 1/2);
% 
% a_ITCG = N*(1+k*sgmf_ksi)*V*lambda_dot + M*(sgmf_abs_sigma-1)*sgmf_ksi*0;
% 
% term = M*(sgmf_abs_sigma-1)*sgmf_ksi;
% 
% if R <10
%     a_ITCG = prev_a_ITCG;
% else
%     a_ITCG = N*(1+k*sgmf_ksi)*V*lambda_dot;
% end

== matlab function ITCG_2D_salvo_attack/CMMAV3/Guidance/MATLAB Function ==
  data: Pos_T_x input; lambda_dot output; Pos_T_y input; Pos_M_x input; Pos_M_y input; psi input; V input; N input; t_go output; sigma_m output; R output
function [lambda_dot, t_go, sigma_m, R] = fcn(Pos_T_x, Pos_T_y, Pos_M_x, Pos_M_y, psi, V, N)
    R2D=180/pi;
    D2R=pi/180;
    % relative parameter
    rTM_x = Pos_T_x - Pos_M_x;
    rTM_y = Pos_T_y - Pos_M_y;
    R=sqrt((rTM_x)^2+(rTM_y)^2);    
    lambda=atan2(rTM_y,rTM_x);
    sigma=psi-lambda;
    sigma_m=abs(mod(sigma+pi, 2*pi)-pi);
    % R_dot=-V*cos(phi);

    % a=1/(2*(N-1));
    % b=1/2;
    % 
    % B1 = integral(@(t) t.^(a-1) .* (1-t).^(b-1), 0, sin(sigma_m)^2, "AbsTol", 1e-10, "RelTol", 1e-4);
    % B2 = beta(a, b);
    % 
    % if isnan(B1)
    %     B1 = 0;
    % end
    % if isnan(B2)
    %     B2 = 0;
    % end
    % 
    % if sigma_m >= 0 && sigma_m < pi/2
    %     t_go = (R / (2*V*(N-1)*sin(sigma_m)^(1/(N-1)))) * B1;
    %     if isinf(t_go) || t_go <= 0.1
    %         t_go = 1e-3;
    %     end
    % elseif sigma_m >= pi/2 && sigma_m <= pi
    %     t_go = (R / (2*V*(N-1)*sin(sigma_m)^(1/(N-1)))) * (2*B2 - B1);
    %     if isinf(t_go) || t_go <= 0.1
    %         t_go = 1e-3;
    %     end
    % else
    %     t_go = 0;
    % end
    
    t_go = R/V*(1+(sigma_m^2/(2*(2*N-1))));

    % command
    lambda_dot = -V*sin(sigma_m)/R;

end

== matlab function ITCG_2D_salvo_attack/CMMAV4/Guidance/ITCG ==
  data: a_ITCG output; lambda_dot input; V input; t_go input; t input; sigma input; ksi output; N input; k input; M input; t_d input; T_god output; R input; prev_a_ITCG input
function [a_ITCG, ksi, T_god]  = fcn(lambda_dot, V, t_go, t, sigma, N, k, M, t_d, R, prev_a_ITCG)


T_god=t_d-t;
ksi=t_go-T_god;

sgmf_ksi = 2*( (1/(1+exp(-10*ksi))) - 1/2);
% sgmf_abs_sigma = 2*( 1/(1+exp(-abs(sigma))) - 1/2);
%
%ITCG command
% a_ITCG = N*(1+k*sign(ksi))*V*theta_dot + M*(sign(abs(phi))-1)*sign(ksi);

if R <10
    a_ITCG = prev_a_ITCG;
else
    a_ITCG = N*(1+k*sgmf_ksi)*V*lambda_dot;
end



% a_ITCG = N*(1+k*sgmf_ksi)*V*lambda_dot + M*(sgmf_abs_sigma-1)*sgmf_ksi;
% function [a_ITCG, ksi, T_god]  = fcn(lambda_dot, V, t_go, t, sigma, N, k, M, t_d, R, prev_a_ITCG)
% 
% T_god = t_d-t;
% ksi = t_go-T_god;
% 
% sigma_deg = sigma * 180/pi;
% 
% sgmf_ksi = 2*( 1/(1+exp(-10*ksi)) - 1/2);
% sgmf_abs_sigma = 2*( 1/(1+exp(-10*abs(sigma_deg))) - 1/2);
% 
% a_ITCG = N*(1+k*sgmf_ksi)*V*lambda_dot + M*(sgmf_abs_sigma-1)*sgmf_ksi*0;
% 
% term = M*(sgmf_abs_sigma-1)*sgmf_ksi;
% 
% if R <10
%     a_ITCG = prev_a_ITCG;
% else
%     a_ITCG = N*(1+k*sgmf_ksi)*V*lambda_dot;
% end

== matlab function ITCG_2D_salvo_attack/CMMAV4/Guidance/MATLAB Function ==
  data: Pos_T_x input; lambda_dot output; Pos_T_y input; Pos_M_x input; Pos_M_y input; psi input; V input; N input; t_go output; sigma_m output; R output
function [lambda_dot, t_go, sigma_m, R] = fcn(Pos_T_x, Pos_T_y, Pos_M_x, Pos_M_y, psi, V, N)
    R2D=180/pi;
    D2R=pi/180;
    % relative parameter
    rTM_x = Pos_T_x - Pos_M_x;
    rTM_y = Pos_T_y - Pos_M_y;
    R=sqrt((rTM_x)^2+(rTM_y)^2);    
    lambda=atan2(rTM_y,rTM_x);
    sigma=psi-lambda;
    sigma_m=abs(mod(sigma+pi, 2*pi)-pi);
    % R_dot=-V*cos(phi);

    % a=1/(2*(N-1));
    % b=1/2;
    % 
    % B1 = integral(@(t) t.^(a-1) .* (1-t).^(b-1), 0, sin(sigma_m)^2, "AbsTol", 1e-10, "RelTol", 1e-4);
    % B2 = beta(a, b);
    % 
    % if isnan(B1)
    %     B1 = 0;
    % end
    % if isnan(B2)
    %     B2 = 0;
    % end
    % 
    % if sigma_m >= 0 && sigma_m < pi/2
    %     t_go = (R / (2*V*(N-1)*sin(sigma_m)^(1/(N-1)))) * B1;
    %     if isinf(t_go) || t_go <= 0.1
    %         t_go = 1e-3;
    %     end
    % elseif sigma_m >= pi/2 && sigma_m <= pi
    %     t_go = (R / (2*V*(N-1)*sin(sigma_m)^(1/(N-1)))) * (2*B2 - B1);
    %     if isinf(t_go) || t_go <= 0.1
    %         t_go = 1e-3;
    %     end
    % else
    %     t_go = 0;
    % end
    
    t_go = R/V*(1+(sigma_m^2/(2*(2*N-1))));

    % command
    lambda_dot = -V*sin(sigma_m)/R;

end

== matlab function ITCG_2D_salvo_attack/Figure/Figure ==
  settings: updateMethod=DISCRETE  sampleTime=0.2
  data: CMMAV1_x input; CMMAV1_y input; CMMAV2_x input; CMMAV2_y input; CMMAV3_x input; CMMAV3_y input; CMMAV4_x input; CMMAV4_y input
function fcn(CMMAV1_x, CMMAV1_y, CMMAV2_x, CMMAV2_y, CMMAV3_x, CMMAV3_y, CMMAV4_x, CMMAV4_y)

persistent data1 timeldx data2 data3 data4 firstFrame filename

if isempty(data1)
    data1 = zeros(100000, 2);  
    timeldx = 1;
end

if isempty(data2)
    data2 = zeros(100000, 2);  
    timeldx = 1;
end

if isempty(data3)
    data3 = zeros(100000, 2);  
    timeldx = 1;
end

if isempty(data4)
    data4 = zeros(100000, 2);  
    timeldx = 1;
end

% GIF 파일 초기화 (첫 실행 시 파일명 설정)
if isempty(firstFrame)
    filename = 'uav_simulation.gif'; % GIF 파일 이름
    firstFrame = true;
end

CMMAV1 = [CMMAV1_x, CMMAV1_y];
CMMAV2 = [CMMAV2_x, CMMAV2_y];
CMMAV3 = [CMMAV3_x, CMMAV3_y];
CMMAV4 = [CMMAV4_x, CMMAV4_y];

data1(timeldx, :) = CMMAV1;
data2(timeldx, :) = CMMAV2;
data3(timeldx, :) = CMMAV3;
data4(timeldx, :) = CMMAV4;

cla; 
grid on;
hold on;

% 이동 경로 그리기
h1 = plot(data1(1:timeldx,1), data1(1:timeldx,2), 'k', 'LineWidth', 1.5);
h2 = plot(data2(1:timeldx,1), data2(1:timeldx,2), 'b', 'LineWidth', 1.5); 
h3 = plot(data3(1:timeldx,1), data3(1:timeldx,2), 'g', 'LineWidth', 1.5); 
h4 = plot(data4(1:timeldx,1), data4(1:timeldx,2), 'm', 'LineWidth', 1.5); 

% 현재 위치를 마커로 표시
plot(CMMAV1_x, CMMAV1_y, 'ko', 'MarkerSize', 8, 'MarkerFaceColor', 'k');
plot(CMMAV2_x, CMMAV2_y, 'bo', 'MarkerSize', 8, 'MarkerFaceColor', 'b');
plot(CMMAV3_x, CMMAV3_y, 'go', 'MarkerSize', 8, 'MarkerFaceColor', 'g');
plot(CMMAV4_x, CMMAV4_y, 'mo', 'MarkerSize', 8, 'MarkerFaceColor', 'm');

% 타겟 포인트 (고정된 원점 0,0)
h5 = plot(0, 0, 'rx', 'MarkerSize', 10, 'LineWidth', 2);

legend([h5, h1, h2, h3, h4], {'Target', 'CMMAV1', 'CMMAV2', 'CMMAV3', 'CMMAV4'}, 'Location', 'NW');

title('2D Impact Time Control Guidance Salvo Attack');
xlabel('X (m)');
ylabel('Y (m)');
xlim([-1000 1000]);
ylim([-1000 1000]);

hold off;

timeldx = timeldx + 1;

end

== matlab function ITCG_2D_salvo_attack/CMMAV1/Guidance/MATLAB Function ==
  data: Pos_T_x input; lambda_dot output; Pos_T_y input; Pos_M_x input; Pos_M_y input; psi input; V input; N input; t_go output; sigma_m output; R output
function [lambda_dot, t_go, sigma_m, R] = fcn(Pos_T_x, Pos_T_y, Pos_M_x, Pos_M_y, psi, V, N)
    R2D=180/pi;
    D2R=pi/180;
    % relative parameter
    rTM_x = Pos_T_x - Pos_M_x;
    rTM_y = Pos_T_y - Pos_M_y;
    R=sqrt((rTM_x)^2+(rTM_y)^2);    
    lambda=atan2(rTM_y,rTM_x);
    sigma=psi-lambda;
    sigma_m=abs(mod(sigma+pi, 2*pi)-pi);
    % R_dot=-V*cos(phi);

    % a=1/(2*(N-1));
    % b=1/2;
    % 
    % B1 = integral(@(t) t.^(a-1) .* (1-t).^(b-1), 0, sin(sigma_m)^2, "AbsTol", 1e-10, "RelTol", 1e-4);
    % B2 = beta(a, b);
    % 
    % if isnan(B1)
    %     B1 = 0;
    % end
    % if isnan(B2)
    %     B2 = 0;
    % end
    % 
    % if sigma_m >= 0 && sigma_m < pi/2
    %     t_go = (R / (2*V*(N-1)*sin(sigma_m)^(1/(N-1)))) * B1;
    %     if isinf(t_go) || t_go <= 0.1
    %         t_go = 1e-3;
    %     end
    % elseif sigma_m >= pi/2 && sigma_m <= pi
    %     t_go = (R / (2*V*(N-1)*sin(sigma_m)^(1/(N-1)))) * (2*B2 - B1);
    %     if isinf(t_go) || t_go <= 0.1
    %         t_go = 1e-3;
    %     end
    % else
    %     t_go = 0;
    % end
    
    t_go = R/V*(1+(sigma_m^2/(2*(2*N-1))));

    % command
    lambda_dot = -V*sin(sigma_m)/R;

end

== matlab function ITCG_2D_salvo_attack/CMMAV1/Guidance/ITCG ==
  data: a_ITCG output; lambda_dot input; V input; t_go input; t input; sigma input; ksi output; N input; k input; M input; t_d input; T_god output; R input; prev_a_ITCG input
function [a_ITCG, ksi, T_god]  = fcn(lambda_dot, V, t_go, t, sigma, N, k, M, t_d, R, prev_a_ITCG)


T_god=t_d-t;
ksi=t_go-T_god;

sgmf_ksi = 2*( (1/(1+exp(-10*ksi))) - 1/2);
% sgmf_abs_sigma = 2*( 1/(1+exp(-abs(sigma))) - 1/2);
%
%ITCG command
% a_ITCG = N*(1+k*sign(ksi))*V*theta_dot + M*(sign(abs(phi))-1)*sign(ksi);

if R <10
    a_ITCG = prev_a_ITCG;
else
    a_ITCG = N*(1+k*sgmf_ksi)*V*lambda_dot;
end



% a_ITCG = N*(1+k*sgmf_ksi)*V*lambda_dot + M*(sgmf_abs_sigma-1)*sgmf_ksi;
% function [a_ITCG, ksi, T_god]  = fcn(lambda_dot, V, t_go, t, sigma, N, k, M, t_d, R, prev_a_ITCG)
% 
% T_god = t_d-t;
% ksi = t_go-T_god;
% 
% sigma_deg = sigma * 180/pi;
% 
% sgmf_ksi = 2*( 1/(1+exp(-10*ksi)) - 1/2);
% sgmf_abs_sigma = 2*( 1/(1+exp(-10*abs(sigma_deg))) - 1/2);
% 
% a_ITCG = N*(1+k*sgmf_ksi)*V*lambda_dot + M*(sgmf_abs_sigma-1)*sgmf_ksi*0;
% 
% term = M*(sgmf_abs_sigma-1)*sgmf_ksi;
% 
% if R <10
%     a_ITCG = prev_a_ITCG;
% else
%     a_ITCG = N*(1+k*sgmf_ksi)*V*lambda_dot;
% end
